simulink model "IEEE9_case"  (R2024b)
settings: Solver=FixedStepAuto  StartTime=0  StopTime=5  FixedStep=1e-7  RelTol=1e-3
values from neighbouring files (symbols this model uses):
  SG_D_1_D = 0.01056    [IEEE9_case_parameters.m]    (also in case1_parameters.m; case2_parameters.m; case3_parameters.m; case4_parameters.m)
  SG_D_1_EnableSaturation = 0    [IEEE9_case_parameters.m]    (also in case1_parameters.m; case2_parameters.m; case3_parameters.m; case4_parameters.m)
  SG_D_1_f0 = 60    [IEEE9_case_parameters.m]    (also in case1_parameters.m; case2_parameters.m; case3_parameters.m; case4_parameters.m)
  SG_D_1_H = 7.5    [IEEE9_case_parameters.m]    (also in case1_parameters.m; case2_parameters.m; case3_parameters.m; case4_parameters.m)
  SG_D_1_K_A = 20    [IEEE9_case_parameters.m]    (also in case1_parameters.m; case2_parameters.m; case3_parameters.m; case4_parameters.m)
  SG_D_1_K_E = 1.000000e+1    (= 10)    [IEEE9_case_parameters.m]    (also in case1_parameters.m; case2_parameters.m; case3_parameters.m; case4_parameters.m)
  SG_D_1_K_F = 2.363    [IEEE9_case_parameters.m]    (also in case1_parameters.m; case2_parameters.m; case3_parameters.m; case4_parameters.m)
  SG_D_1_K_s = 0.5    [IEEE9_case_parameters.m]    (also in case1_parameters.m = 5; case2_parameters.m = 5; case3_parameters.m = 5; case4_parameters.m = 5)
  SG_D_1_R_a = 0.001088    [IEEE9_case_parameters.m]    (also in case1_parameters.m; case2_parameters.m; case3_parameters.m; case4_parameters.m)
  SG_D_1_S_A = 1    [IEEE9_case_parameters.m]    (also in case1_parameters.m; case2_parameters.m; case3_parameters.m; case4_parameters.m)
  SG_D_1_S_B = 0.103    [IEEE9_case_parameters.m]    (also in case1_parameters.m; case2_parameters.m; case3_parameters.m; case4_parameters.m)
  SG_D_1_S_N = 10.659857    [IEEE9_case_parameters.m]    (also in case1_parameters.m; case2_parameters.m; case3_parameters.m; case4_parameters.m)
  SG_D_1_SpeedPara = 200    [IEEE9_case_parameters.m]    (also in case1_parameters.m; case2_parameters.m; case3_parameters.m; case4_parameters.m)
  SG_D_1_T_0 = 0.720173    [IEEE9_case_parameters.m]    (also in case1_parameters.m = 0.755522; case2_parameters.m = 0.808931; case3_parameters.m = 0.869402; case4_parameters.m = 0.729316)
  SG_D_1_T_1 = 0.3    [IEEE9_case_parameters.m]    (also in case1_parameters.m; case2_parameters.m; case3_parameters.m; case4_parameters.m)
  SG_D_1_T_2 = 0.05    [IEEE9_case_parameters.m]    (also in case1_parameters.m; case2_parameters.m; case3_parameters.m; case4_parameters.m)
  SG_D_1_T_3 = 0.02    [IEEE9_case_parameters.m]    (also in case1_parameters.m; case2_parameters.m; case3_parameters.m; case4_parameters.m)
  SG_D_1_T_4 = 0.005    [IEEE9_case_parameters.m]    (also in case1_parameters.m; case2_parameters.m; case3_parameters.m; case4_parameters.m)
  SG_D_1_T_A = 0.02    [IEEE9_case_parameters.m]    (also in case1_parameters.m; case2_parameters.m; case3_parameters.m; case4_parameters.m)
  SG_D_1_T_dd = 8.000000e+0    (= 8)    [IEEE9_case_parameters.m]    (also in case1_parameters.m; case2_parameters.m; case3_parameters.m; case4_parameters.m)
  SG_D_1_T_ddd = 0.04    [IEEE9_case_parameters.m]    (also in case1_parameters.m; case2_parameters.m; case3_parameters.m; case4_parameters.m)
  SG_D_1_T_E = 0.314    [IEEE9_case_parameters.m]    (also in case1_parameters.m; case2_parameters.m; case3_parameters.m; case4_parameters.m)
  SG_D_1_T_F = 0.35    [IEEE9_case_parameters.m]    (also in case1_parameters.m; case2_parameters.m; case3_parameters.m; case4_parameters.m)
  SG_D_1_T_qd = 0.8    [IEEE9_case_parameters.m]    (also in case1_parameters.m; case2_parameters.m; case3_parameters.m; case4_parameters.m)
  SG_D_1_T_qdd = 0.02    [IEEE9_case_parameters.m]    (also in case1_parameters.m; case2_parameters.m; case3_parameters.m; case4_parameters.m)
  SG_D_1_T_speed = 0.1    [IEEE9_case_parameters.m]    (also in case1_parameters.m = 200; case2_parameters.m = 200; case3_parameters.m = 200; case4_parameters.m = 200)
  SG_D_1_T_w = 0.5    [IEEE9_case_parameters.m]    (also in case1_parameters.m; case2_parameters.m; case3_parameters.m; case4_parameters.m)
  SG_D_1_V_ref = 1.990276    [IEEE9_case_parameters.m]    (also in case1_parameters.m = 2.042296; case2_parameters.m = 2.051388; case3_parameters.m = 2.089584; case4_parameters.m = 2.01845)
  SG_D_1_w_ref = 376.991118    [IEEE9_case_parameters.m]    (also in case1_parameters.m; case2_parameters.m; case3_parameters.m; case4_parameters.m)
  SG_D_1_wb = 6.000000e+1    (= 60)    [IEEE9_case_parameters.m]    (also in case1_parameters.m; case2_parameters.m; case3_parameters.m; case4_parameters.m)
  SG_D_1_x_d = 1.9    [IEEE9_case_parameters.m]    (also in case1_parameters.m; case2_parameters.m; case3_parameters.m; case4_parameters.m)
  SG_D_1_x_dd = 0.302    [IEEE9_case_parameters.m]    (also in case1_parameters.m; case2_parameters.m; case3_parameters.m; case4_parameters.m)
  SG_D_1_x_ddd = 0.204    [IEEE9_case_parameters.m]    (also in case1_parameters.m; case2_parameters.m; case3_parameters.m; case4_parameters.m)
  SG_D_1_x_l = 0.05    [IEEE9_case_parameters.m]    (also in case1_parameters.m; case2_parameters.m; case3_parameters.m; case4_parameters.m)
  SG_D_1_x_q = 1.3    [IEEE9_case_parameters.m]    (also in case1_parameters.m; case2_parameters.m; case3_parameters.m; case4_parameters.m)
  SG_D_1_x_qd = 0.5    [IEEE9_case_parameters.m]    (also in case1_parameters.m; case2_parameters.m; case3_parameters.m; case4_parameters.m)
  SG_D_1_x_qdd = 0.3    [IEEE9_case_parameters.m]    (also in case1_parameters.m; case2_parameters.m; case3_parameters.m; case4_parameters.m)
  SG_D_2_D = 0.02    [IEEE9_case_parameters.m]    (also in case1_parameters.m; case2_parameters.m; case3_parameters.m; case4_parameters.m)
  SG_D_2_EnableSaturation = 0    [IEEE9_case_parameters.m]    (also in case1_parameters.m; case2_parameters.m; case3_parameters.m; case4_parameters.m)
  SG_D_2_f0 = 60    [IEEE9_case_parameters.m]    (also in case1_parameters.m; case2_parameters.m; case3_parameters.m; case4_parameters.m)
  SG_D_2_H = 8.000000e+0    (= 8)    [IEEE9_case_parameters.m]    (also in case1_parameters.m; case2_parameters.m; case3_parameters.m; case4_parameters.m)
  SG_D_2_K_A = 20    [IEEE9_case_parameters.m]    (also in case1_parameters.m; case2_parameters.m; case3_parameters.m; case4_parameters.m)
  SG_D_2_K_E = 1.000000e+1    (= 10)    [IEEE9_case_parameters.m]    (also in case1_parameters.m; case2_parameters.m; case3_parameters.m; case4_parameters.m)
  SG_D_2_K_F = 2.363    [IEEE9_case_parameters.m]    (also in case1_parameters.m; case2_parameters.m; case3_parameters.m; case4_parameters.m)
  SG_D_2_K_s = 0.5    [IEEE9_case_parameters.m]    (also in case1_parameters.m = 4; case2_parameters.m = 4; case3_parameters.m = 4; case4_parameters.m = 4)
  SG_D_2_R_a = 0.001088    [IEEE9_case_parameters.m]    (also in case1_parameters.m; case2_parameters.m; case3_parameters.m; case4_parameters.m)
  SG_D_2_S_A = 1    [IEEE9_case_parameters.m]    (also in case1_parameters.m; case2_parameters.m; case3_parameters.m; case4_parameters.m)
  SG_D_2_S_B = 0.103    [IEEE9_case_parameters.m]    (also in case1_parameters.m; case2_parameters.m; case3_parameters.m; case4_parameters.m)
  SG_D_2_S_N = 10.659857    [IEEE9_case_parameters.m]    (also in case1_parameters.m; case2_parameters.m; case3_parameters.m; case4_parameters.m)
  SG_D_2_SpeedPara = 200    [IEEE9_case_parameters.m]    (also in case1_parameters.m; case2_parameters.m; case3_parameters.m; case4_parameters.m)
  SG_D_2_T_0 = 1.632913    [IEEE9_case_parameters.m]    (also in case1_parameters.m = 1.632925; case2_parameters.m = 1.632915; case3_parameters.m = 1.632914; case4_parameters.m = 1.632927)
  SG_D_2_T_1 = 0.2    [IEEE9_case_parameters.m]    (also in case1_parameters.m; case2_parameters.m; case3_parameters.m; case4_parameters.m)
  SG_D_2_T_2 = 0.05    [IEEE9_case_parameters.m]    (also in case1_parameters.m; case2_parameters.m; case3_parameters.m; case4_parameters.m)
  SG_D_2_T_3 = 0.02    [IEEE9_case_parameters.m]    (also in case1_parameters.m; case2_parameters.m; case3_parameters.m; case4_parameters.m)
  SG_D_2_T_4 = 0.005    [IEEE9_case_parameters.m]    (also in case1_parameters.m; case2_parameters.m; case3_parameters.m; case4_parameters.m)
  SG_D_2_T_A = 0.02    [IEEE9_case_parameters.m]    (also in case1_parameters.m; case2_parameters.m; case3_parameters.m; case4_parameters.m)
  SG_D_2_T_dd = 7.9    [IEEE9_case_parameters.m]    (also in case1_parameters.m; case2_parameters.m; case3_parameters.m; case4_parameters.m)
  SG_D_2_T_ddd = 0.04    [IEEE9_case_parameters.m]    (also in case1_parameters.m; case2_parameters.m; case3_parameters.m; case4_parameters.m)
  SG_D_2_T_E = 0.314    [IEEE9_case_parameters.m]    (also in case1_parameters.m; case2_parameters.m; case3_parameters.m; case4_parameters.m)
  SG_D_2_T_F = 0.35    [IEEE9_case_parameters.m]    (also in case1_parameters.m; case2_parameters.m; case3_parameters.m; case4_parameters.m)
  SG_D_2_T_qd = 0.8    [IEEE9_case_parameters.m]    (also in case1_parameters.m; case2_parameters.m; case3_parameters.m; case4_parameters.m)
  SG_D_2_T_qdd = 0.015    [IEEE9_case_parameters.m]    (also in case1_parameters.m; case2_parameters.m; case3_parameters.m; case4_parameters.m)
  SG_D_2_T_speed = 0.1    [IEEE9_case_parameters.m]    (also in case1_parameters.m = 150; case2_parameters.m = 150; case3_parameters.m = 150; case4_parameters.m = 150)
  SG_D_2_T_w = 0.35    [IEEE9_case_parameters.m]    (also in case1_parameters.m; case2_parameters.m; case3_parameters.m; case4_parameters.m)
  SG_D_2_V_ref = 2.58547    [IEEE9_case_parameters.m]    (also in case1_parameters.m = 2.597896; case2_parameters.m = 2.587136; case3_parameters.m = 2.586042; case4_parameters.m = 2.599679)
  SG_D_2_w_ref = 376.991118    [IEEE9_case_parameters.m]    (also in case1_parameters.m; case2_parameters.m; case3_parameters.m; case4_parameters.m)
  SG_D_2_wb = 6.000000e+1    (= 60)    [IEEE9_case_parameters.m]    (also in case1_parameters.m; case2_parameters.m; case3_parameters.m; case4_parameters.m)
  SG_D_2_x_d = 1.8    [IEEE9_case_parameters.m]    (also in case1_parameters.m; case2_parameters.m; case3_parameters.m; case4_parameters.m)
  SG_D_2_x_dd = 0.302    [IEEE9_case_parameters.m]    (also in case1_parameters.m; case2_parameters.m; case3_parameters.m; case4_parameters.m)
  SG_D_2_x_ddd = 0.204    [IEEE9_case_parameters.m]    (also in case1_parameters.m; case2_parameters.m; case3_parameters.m; case4_parameters.m)
  SG_D_2_x_l = 0.05    [IEEE9_case_parameters.m]    (also in case1_parameters.m; case2_parameters.m; case3_parameters.m; case4_parameters.m)
  SG_D_2_x_q = 1.25    [IEEE9_case_parameters.m]    (also in case1_parameters.m; case2_parameters.m; case3_parameters.m; case4_parameters.m)
  SG_D_2_x_qd = 0.5    [IEEE9_case_parameters.m]    (also in case1_parameters.m; case2_parameters.m; case3_parameters.m; case4_parameters.m)
  SG_D_2_x_qdd = 0.3    [IEEE9_case_parameters.m]    (also in case1_parameters.m; case2_parameters.m; case3_parameters.m; case4_parameters.m)
  SG_D_3_D = 0.02    [IEEE9_case_parameters.m]    (also in case1_parameters.m; case2_parameters.m; case3_parameters.m; case4_parameters.m)
  SG_D_3_EnableSaturation = 0    [IEEE9_case_parameters.m]    (also in case1_parameters.m; case2_parameters.m; case3_parameters.m; case4_parameters.m)
  SG_D_3_f0 = 60    [IEEE9_case_parameters.m]    (also in case1_parameters.m; case2_parameters.m; case3_parameters.m; case4_parameters.m)
  SG_D_3_H = 7.7    [IEEE9_case_parameters.m]    (also in case1_parameters.m; case2_parameters.m; case3_parameters.m; case4_parameters.m)
  SG_D_3_K_A = 20    [IEEE9_case_parameters.m]    (also in case1_parameters.m; case2_parameters.m; case3_parameters.m; case4_parameters.m)
  SG_D_3_K_E = 1.000000e+1    (= 10)    [IEEE9_case_parameters.m]    (also in case1_parameters.m; case2_parameters.m; case3_parameters.m; case4_parameters.m)
  SG_D_3_K_F = 2.363    [IEEE9_case_parameters.m]    (also in case1_parameters.m; case2_parameters.m; case3_parameters.m; case4_parameters.m)
  SG_D_3_K_s = 0.2    [IEEE9_case_parameters.m]    (also in case1_parameters.m = 2; case2_parameters.m = 2; case3_parameters.m = 2; case4_parameters.m = 2)
  SG_D_3_R_a = 0.001088    [IEEE9_case_parameters.m]    (also in case1_parameters.m; case2_parameters.m; case3_parameters.m; case4_parameters.m)
  SG_D_3_S_A = 1    [IEEE9_case_parameters.m]    (also in case1_parameters.m; case2_parameters.m; case3_parameters.m; case4_parameters.m)
  SG_D_3_S_B = 0.103    [IEEE9_case_parameters.m]    (also in case1_parameters.m; case2_parameters.m; case3_parameters.m; case4_parameters.m)
  SG_D_3_S_N = 10.659857    [IEEE9_case_parameters.m]    (also in case1_parameters.m; case2_parameters.m; case3_parameters.m; case4_parameters.m)
  SG_D_3_SpeedPara = 200    [IEEE9_case_parameters.m]    (also in case1_parameters.m; case2_parameters.m; case3_parameters.m; case4_parameters.m)
  SG_D_3_T_0 = 0.850788    [IEEE9_case_parameters.m]    (also in case1_parameters.m = 0.850786; case2_parameters.m = 0.850787; case3_parameters.m; case4_parameters.m = 0.850786)
  SG_D_3_T_1 = 0.2    [IEEE9_case_parameters.m]    (also in case1_parameters.m; case2_parameters.m; case3_parameters.m; case4_parameters.m)
  SG_D_3_T_2 = 0.05    [IEEE9_case_parameters.m]    (also in case1_parameters.m; case2_parameters.m; case3_parameters.m; case4_parameters.m)
  SG_D_3_T_3 = 0.02    [IEEE9_case_parameters.m]    (also in case1_parameters.m; case2_parameters.m; case3_parameters.m; case4_parameters.m)
  SG_D_3_T_4 = 0.005    [IEEE9_case_parameters.m]    (also in case1_parameters.m; case2_parameters.m; case3_parameters.m; case4_parameters.m)
  SG_D_3_T_A = 0.02    [IEEE9_case_parameters.m]    (also in case1_parameters.m; case2_parameters.m; case3_parameters.m; case4_parameters.m)
  SG_D_3_T_dd = 8.1    [IEEE9_case_parameters.m]    (also in case1_parameters.m; case2_parameters.m; case3_parameters.m; case4_parameters.m)
  SG_D_3_T_ddd = 0.04    [IEEE9_case_parameters.m]    (also in case1_parameters.m; case2_parameters.m; case3_parameters.m; case4_parameters.m)
  SG_D_3_T_E = 0.314    [IEEE9_case_parameters.m]    (also in case1_parameters.m; case2_parameters.m; case3_parameters.m; case4_parameters.m)
  SG_D_3_T_F = 0.35    [IEEE9_case_parameters.m]    (also in case1_parameters.m; case2_parameters.m; case3_parameters.m; case4_parameters.m)
  SG_D_3_T_qd = 0.8    [IEEE9_case_parameters.m]    (also in case1_parameters.m; case2_parameters.m; case3_parameters.m; case4_parameters.m)
  SG_D_3_T_qdd = 0.015    [IEEE9_case_parameters.m]    (also in case1_parameters.m; case2_parameters.m; case3_parameters.m; case4_parameters.m)
  SG_D_3_T_speed = 0.1    [IEEE9_case_parameters.m]    (also in case1_parameters.m = 180; case2_parameters.m = 180; case3_parameters.m = 180; case4_parameters.m = 180)
  SG_D_3_T_w = 0.4    [IEEE9_case_parameters.m]    (also in case1_parameters.m; case2_parameters.m; case3_parameters.m; case4_parameters.m)
  SG_D_3_V_ref = 1.892727    [IEEE9_case_parameters.m]    (also in case1_parameters.m = 1.906439; case2_parameters.m = 1.895535; case3_parameters.m = 1.892105; case4_parameters.m = 1.906598)
  SG_D_3_w_ref = 376.991118    [IEEE9_case_parameters.m]    (also in case1_parameters.m; case2_parameters.m; case3_parameters.m; case4_parameters.m)
  SG_D_3_wb = 6.000000e+1    (= 60)    [IEEE9_case_parameters.m]    (also in case1_parameters.m; case2_parameters.m; case3_parameters.m; case4_parameters.m)
  SG_D_3_x_d = 1.85    [IEEE9_case_parameters.m]    (also in case1_parameters.m; case2_parameters.m; case3_parameters.m; case4_parameters.m)
  SG_D_3_x_dd = 0.302    [IEEE9_case_parameters.m]    (also in case1_parameters.m; case2_parameters.m; case3_parameters.m; case4_parameters.m)
  SG_D_3_x_ddd = 0.204    [IEEE9_case_parameters.m]    (also in case1_parameters.m; case2_parameters.m; case3_parameters.m; case4_parameters.m)
  SG_D_3_x_l = 0.05    [IEEE9_case_parameters.m]    (also in case1_parameters.m; case2_parameters.m; case3_parameters.m; case4_parameters.m)
  SG_D_3_x_q = 1.2    [IEEE9_case_parameters.m]    (also in case1_parameters.m; case2_parameters.m; case3_parameters.m; case4_parameters.m)
  SG_D_3_x_qd = 0.5    [IEEE9_case_parameters.m]    (also in case1_parameters.m; case2_parameters.m; case3_parameters.m; case4_parameters.m)
  SG_D_3_x_qdd = 0.3    [IEEE9_case_parameters.m]    (also in case1_parameters.m; case2_parameters.m; case3_parameters.m; case4_parameters.m)
(part 6 of 12)

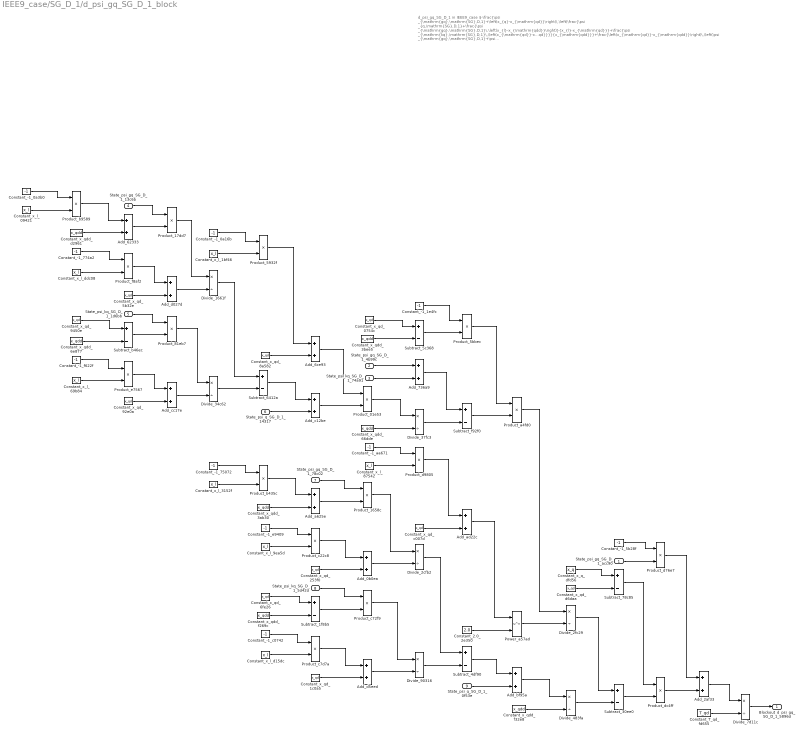
== system IEEE9_case/SG_D_1/d_psi_gq_SG_D_1_block ==
  note: d_psi_gq_SG_D_1 in IEEE9_case
      | $-\frac{\psi _{\mathrm{gq},\mathrm{SG},D,1}+\left(x_{q}-x_{\mathrm{qd}}\right)\,\left(\frac{\psi _{q,\mathrm{SG},D,1}+\frac{\psi _{\mathrm{gq},\mathrm{SG},D,1}\,\left(x_{l}-x_{\mathrm{qdd}}\right)}{x_{l}-x_{\mathrm{qd}}}+\frac{\psi _{\mathrm{kq},\mathrm{SG},D,1}\,\left(x_{\mathrm{qd}}-x_{\mathrm{qdd}}\right)}{x_{l}-x_{\mathrm{qd}}}}{x_{\mathrm{qdd}}}+\frac{\left(x_{\mathrm{qd}}-x_{\mathrm{qdd}}\right)\,\left(\psi _{\mathrm{gq},\mathrm{SG},D,1}+\psi _{\mathrm{kq},\mathrm{SG},D,1}+\frac{\left(x_{l}-x_{\mathrm{qd}}\right)\,\left(\psi _{q,\mathrm{SG},D,1}+\frac{\psi _{\mathrm{gq},\mathrm{SG},D,1}\,\left(x_{l}-x_{\mathrm{qdd}}\right)}{x_{l}-x_{\mathrm{qd}}}+\frac{\psi _{\mathrm{kq},\mathrm{SG},D,1}\,\left(x_{\mathrm{qd}}-x_{\mathrm{qdd}}\right)}{x_{l}-x_{\mathrm{qd}}}\right)}{x_{\mathrm{qdd}}}\right)}{{\left(x_{l}-x_{\mathrm{qd}}\right)}^2}\right)}{T_{\mathrm{qd}}}$
      | Automatically generated on 2025-11-01 08:47:44 .
  State_psi_gq_SG_D_1_acc90 : Inport
  State_psi_gq_SG_D_1_4b99c : Inport  Port=2
  State_psi_kq_SG_D_1_74a91 : Inport  Port=3
  State_psi_gq_SG_D_1_13c6b : Inport  Port=4
  State_psi_kq_SG_D_1_1d6bb : Inport  Port=5
  State_psi_q_SG_D_1_14317 : Inport  Port=6
  State_psi_gq_SG_D_1_78c02 : Inport  Port=7
  State_psi_kq_SG_D_1_5d42d : Inport  Port=8
  State_psi_q_SG_D_1_0f53e : Inport  Port=9
  Add_0b0ea : Sum
  Add_2af33 : Sum
  Add_62333 : Sum
  Add_6ce93 : Sum
  Add_736a9 : Sum
  Add_a625e : Sum
  Add_ad22c : Sum
  Add_bf95a : Sum
  Add_c12be : Sum
  Add_cc17e : Sum
  Add_d027d : Sum
  Add_d5eed : Sum
  Constant_-1_0a16b : Constant  Value=-1
  Constant_-1_0a3b0 : Constant  Value=-1
  Constant_-1_1e4fc : Constant  Value=-1
  Constant_-1_5b28f : Constant  Value=-1
  Constant_-1_75072 : Constant  Value=-1
  Constant_-1_774a2 : Constant  Value=-1
  Constant_-1_aa671 : Constant  Value=-1
  Constant_-1_c0742 : Constant  Value=-1
  Constant_-1_e9409 : Constant  Value=-1
  Constant_-1_f622f : Constant  Value=-1
  Constant_2.0_2e350 : Constant  Value=2.0
  Constant_T_qd_fd655 : Constant  Value=T_qd
  Constant_x_l_09421 : Constant  Value=x_l
  Constant_x_l_1bf46 : Constant  Value=x_l
  Constant_x_l_3152f : Constant  Value=x_l
  Constant_x_l_69b84 : Constant  Value=x_l
  Constant_x_l_87542 : Constant  Value=x_l
  Constant_x_l_9ea5d : Constant  Value=x_l
  Constant_x_l_d15dc : Constant  Value=x_l
  Constant_x_l_ddc08 : Constant  Value=x_l
  Constant_x_q_dfd56 : Constant  Value=x_q
  Constant_x_qd_0754c : Constant  Value=x_qd
  Constant_x_qd_1c0a5 : Constant  Value=x_qd
  Constant_x_qd_253f0 : Constant  Value=x_qd
  Constant_x_qd_5b32e : Constant  Value=x_qd
  Constant_x_qd_6fe26 : Constant  Value=x_qd
  Constant_x_qd_8a582 : Constant  Value=x_qd
  Constant_x_qd_92e0a : Constant  Value=x_qd
  Constant_x_qd_9450e : Constant  Value=x_qd
  Constant_x_qd_c007d : Constant  Value=x_qd
  Constant_x_qd_d6daa : Constant  Value=x_qd
  Constant_x_qdd_3ab30 : Constant  Value=x_qdd
  Constant_x_qdd_3bee5 : Constant  Value=x_qdd
  Constant_x_qdd_66dde : Constant  Value=x_qdd
  Constant_x_qdd_6e877 : Constant  Value=x_qdd
  Constant_x_qdd_d2961 : Constant  Value=x_qdd
  Constant_x_qdd_f269c : Constant  Value=x_qdd
  Constant_x_qdd_f32e8 : Constant  Value=x_qdd
  Divide_1661f : Product  Inputs=*/
  Divide_2cfb2 : Product  Inputs=*/
  Divide_2fc29 : Product  Inputs=*/
  Divide_34c62 : Product  Inputs=*/
  Divide_37fc3 : Product  Inputs=*/
  Divide_483fa : Product  Inputs=*/
  Divide_7d11c : Product  Inputs=*/
  Divide_90316 : Product  Inputs=*/
  Power_a57ad : Math  Operator=pow
  Product_01e53 : Product
  Product_1658c : Product
  Product_17dd7 : Product
  Product_5932f : Product
  Product_5bbec : Product
  Product_81eb7 : Product
  Product_a4fd0 : Product
  Product_b435c : Product
  Product_b9589 : Product
  Product_c22c8 : Product
  Product_c72f9 : Product
  Product_c7d7a : Product
  Product_d76e7 : Product
  Product_d9805 : Product
  Product_dc4ff : Product
  Product_e7567 : Product
  Product_f8af2 : Product
  Subtract_1f8b5 : Sum  Inputs=+-
  Subtract_30ee0 : Sum  Inputs=+-
  Subtract_4df90 : Sum  Inputs=+-
  Subtract_5c368 : Sum  Inputs=+-
  Subtract_6412a : Sum  Inputs=+-
  Subtract_78c85 : Sum  Inputs=+-
  Subtract_b46ec : Sum  Inputs=+-
  Subtract_f92f0 : Sum  Inputs=+-
  Blockout_d_psi_gq_SG_D_1_5896d : Outport
  wires:
  State_psi_gq_SG_D_1_13c6b/1 -> Product_17dd7/1
  Constant_-1_774a2/1 -> Product_f8af2/1
  Divide_1661f/1 -> Subtract_6412a/1
  Add_d027d/1 -> Divide_1661f/2
  Product_b9589/1 -> Add_62333/1
  Constant_x_qd_8a582/1 -> Add_6ce93/2
  Constant_-1_0a3b0/1 -> Product_b9589/1
  Constant_x_qdd_d2961/1 -> Add_62333/2
  Constant_x_l_ddc08/1 -> Product_f8af2/2
  Constant_x_l_09421/1 -> Product_b9589/2
  Constant_-1_f622f/1 -> Product_e7567/1
  Constant_x_qd_9450e/1 -> Subtract_b46ec/1
  Constant_x_qdd_66dde/1 -> Divide_37fc3/2
  Constant_x_l_69b84/1 -> Product_e7567/2
  Constant_x_qdd_6e877/1 -> Subtract_b46ec/2
  Subtract_6412a/1 -> Add_c12be/1
  Add_62333/1 -> Product_17dd7/2
  Product_17dd7/1 -> Divide_1661f/1
  Product_f8af2/1 -> Add_d027d/1
  Constant_x_qd_5b32e/1 -> Add_d027d/2
  State_psi_kq_SG_D_1_1d6bb/1 -> Product_81eb7/1
  Product_e7567/1 -> Add_cc17e/1
  Subtract_b46ec/1 -> Product_81eb7/2
  Constant_x_qd_92e0a/1 -> Add_cc17e/2
  Product_81eb7/1 -> Divide_34c62/1
  Add_cc17e/1 -> Divide_34c62/2
  Constant_-1_1e4fc/1 -> Product_5bbec/1
  Constant_-1_0a16b/1 -> Product_5932f/1
  Add_0b0ea/1 -> Divide_2cfb2/2
  Product_c7d7a/1 -> Add_d5eed/1
  Subtract_1f8b5/1 -> Product_c72f9/2
  Constant_x_l_1bf46/1 -> Product_5932f/2
  Divide_34c62/1 -> Subtract_6412a/2
  Subtract_78c85/1 -> Product_dc4ff/1
  Constant_-1_aa671/1 -> Product_d9805/1
  Constant_-1_75072/1 -> Product_b435c/1
  Constant_x_l_87542/1 -> Product_d9805/2
  Constant_x_l_3152f/1 -> Product_b435c/2
  Constant_x_qd_253f0/1 -> Add_0b0ea/2
  Product_5932f/1 -> Add_6ce93/1
  State_psi_q_SG_D_1_14317/1 -> Add_c12be/2
  Product_b435c/1 -> Add_a625e/1
  Constant_x_qdd_3ab30/1 -> Add_a625e/2
  Constant_-1_e9409/1 -> Product_c22c8/1
  Constant_x_qd_1c0a5/1 -> Add_d5eed/2
  Add_6ce93/1 -> Product_01e53/1
  Constant_x_l_9ea5d/1 -> Product_c22c8/2
  Constant_-1_c0742/1 -> Product_c7d7a/1
  Constant_x_qd_6fe26/1 -> Subtract_1f8b5/1
  Product_01e53/1 -> Divide_37fc3/1
  Constant_x_l_d15dc/1 -> Product_c7d7a/2
  Divide_2fc29/1 -> Subtract_30ee0/1
  Constant_x_qdd_f269c/1 -> Subtract_1f8b5/2
  Add_c12be/1 -> Product_01e53/2
  State_psi_gq_SG_D_1_78c02/1 -> Product_1658c/1
  Add_a625e/1 -> Product_1658c/2
  Product_c22c8/1 -> Add_0b0ea/1
  State_psi_kq_SG_D_1_5d42d/1 -> Product_c72f9/1
  Add_d5eed/1 -> Divide_90316/2
  State_psi_gq_SG_D_1_4b99c/1 -> Add_736a9/1
  Constant_x_qd_0754c/1 -> Subtract_5c368/1
  Constant_x_qdd_3bee5/1 -> Subtract_5c368/2
  Product_c72f9/1 -> Divide_90316/1
  State_psi_kq_SG_D_1_74a91/1 -> Add_736a9/2
  Product_1658c/1 -> Divide_2cfb2/1
  Subtract_5c368/1 -> Product_5bbec/2
  Add_736a9/1 -> Subtract_f92f0/1
  Divide_37fc3/1 -> Subtract_f92f0/2
  Product_d9805/1 -> Add_ad22c/1
  Constant_x_qd_c007d/1 -> Add_ad22c/2
  Divide_2cfb2/1 -> Subtract_4df90/1
  Divide_90316/1 -> Subtract_4df90/2
  Product_5bbec/1 -> Product_a4fd0/1
  Subtract_f92f0/1 -> Product_a4fd0/2
  Add_ad22c/1 -> Power_a57ad/1
  Constant_2.0_2e350/1 -> Power_a57ad/2
  Subtract_4df90/1 -> Add_bf95a/1
  State_psi_q_SG_D_1_0f53e/1 -> Add_bf95a/2
  Product_a4fd0/1 -> Divide_2fc29/1
  Power_a57ad/1 -> Divide_2fc29/2
  Add_bf95a/1 -> Divide_483fa/1
  Constant_x_qdd_f32e8/1 -> Divide_483fa/2
  Constant_x_q_dfd56/1 -> Subtract_78c85/1
  Constant_x_qd_d6daa/1 -> Subtract_78c85/2
  Divide_483fa/1 -> Subtract_30ee0/2
  Constant_-1_5b28f/1 -> Product_d76e7/1
  State_psi_gq_SG_D_1_acc90/1 -> Product_d76e7/2
  Subtract_30ee0/1 -> Product_dc4ff/2
  Product_d76e7/1 -> Add_2af33/1
  Product_dc4ff/1 -> Add_2af33/2
  Add_2af33/1 -> Divide_7d11c/1
  Constant_T_qd_fd655/1 -> Divide_7d11c/2
  Divide_7d11c/1 -> Blockout_d_psi_gq_SG_D_1_5896d/1

== system IEEE9_case/SG_D_1/d_psi_kq_SG_D_1_block ==
  note: d_psi_kq_SG_D_1 in IEEE9_case
      | $-\frac{\psi _{\mathrm{gq},\mathrm{SG},D,1}+\psi _{\mathrm{kq},\mathrm{SG},D,1}+\frac{\left(x_{l}-x_{\mathrm{qd}}\right)\,\left(\psi _{q,\mathrm{SG},D,1}+\frac{\psi _{\mathrm{gq},\mathrm{SG},D,1}\,\left(x_{l}-x_{\mathrm{qdd}}\right)}{x_{l}-x_{\mathrm{qd}}}+\frac{\psi _{\mathrm{kq},\mathrm{SG},D,1}\,\left(x_{\mathrm{qd}}-x_{\mathrm{qdd}}\right)}{x_{l}-x_{\mathrm{qd}}}\right)}{x_{\mathrm{qdd}}}}{T_{\mathrm{qdd}}}$
      | Automatically generated on 2025-11-01 08:47:48 .
  State_psi_gq_SG_D_1_49d8b : Inport
  State_psi_kq_SG_D_1_01b22 : Inport  Port=2
  State_psi_gq_SG_D_1_47bd3 : Inport  Port=3
  State_psi_kq_SG_D_1_dfcd5 : Inport  Port=4
  State_psi_q_SG_D_1_68fd5 : Inport  Port=5
  Add_084c3 : Sum
  Add_2c012 : Sum
  Add_2f0c8 : Sum
  Add_49d96 : Sum
  Add_85ea5 : Sum
  Add_fad76 : Sum
  Constant_-1_72ab9 : Constant  Value=-1
  Constant_-1_92c62 : Constant  Value=-1
  Constant_-1_ac321 : Constant  Value=-1
  Constant_-1_b5108 : Constant  Value=-1
  Constant_-1_c3780 : Constant  Value=-1
  Constant_T_qdd_57beb : Constant  Value=T_qdd
  Constant_x_l_311b0 : Constant  Value=x_l
  Constant_x_l_3981a : Constant  Value=x_l
  Constant_x_l_62966 : Constant  Value=x_l
  Constant_x_l_98c38 : Constant  Value=x_l
  Constant_x_qd_3af05 : Constant  Value=x_qd
  Constant_x_qd_6fbee : Constant  Value=x_qd
  Constant_x_qd_a7fbb : Constant  Value=x_qd
  Constant_x_qd_cbc91 : Constant  Value=x_qd
  Constant_x_qdd_0a2c9 : Constant  Value=x_qdd
  Constant_x_qdd_25906 : Constant  Value=x_qdd
  Constant_x_qdd_e3520 : Constant  Value=x_qdd
  Divide_1a1ce : Product  Inputs=*/
  Divide_5f60d : Product  Inputs=*/
  Divide_7895a : Product  Inputs=*/
  Divide_f11d6 : Product  Inputs=*/
  Product_0ea38 : Product
  Product_3e32f : Product
  Product_40f55 : Product
  Product_67d0d : Product
  Product_b6550 : Product
  Product_c92d2 : Product
  Product_cd562 : Product
  Product_d66a1 : Product
  Subtract_0bd57 : Sum  Inputs=+-
  Subtract_bee95 : Sum  Inputs=+-
  Subtract_e02f6 : Sum  Inputs=+-
  Blockout_d_psi_kq_SG_D_1_c4f81 : Outport
  wires:
  Product_d66a1/1 -> Add_084c3/1
  Constant_-1_72ab9/1 -> Product_d66a1/1
  Constant_x_l_62966/1 -> Product_d66a1/2
  Constant_x_qdd_0a2c9/1 -> Add_084c3/2
  Constant_-1_92c62/1 -> Product_c92d2/1
  Constant_x_qd_6fbee/1 -> Subtract_e02f6/1
  Constant_x_qd_cbc91/1 -> Add_49d96/2
  Constant_-1_ac321/1 -> Product_40f55/1
  Constant_x_l_98c38/1 -> Product_c92d2/2
  Constant_x_qdd_25906/1 -> Subtract_e02f6/2
  Constant_x_qd_a7fbb/1 -> Add_2f0c8/2
  Constant_x_l_3981a/1 -> Product_40f55/2
  Subtract_bee95/1 -> Add_fad76/1
  Product_67d0d/1 -> Subtract_bee95/1
  State_psi_gq_SG_D_1_47bd3/1 -> Product_cd562/1
  Add_084c3/1 -> Product_cd562/2
  Product_40f55/1 -> Add_85ea5/1
  Constant_x_qd_3af05/1 -> Add_85ea5/2
  State_psi_kq_SG_D_1_dfcd5/1 -> Product_0ea38/1
  Product_c92d2/1 -> Add_2f0c8/1
  Subtract_e02f6/1 -> Product_0ea38/2
  Product_cd562/1 -> Divide_7895a/1
  Add_85ea5/1 -> Divide_7895a/2
  Product_0ea38/1 -> Divide_f11d6/1
  Add_2f0c8/1 -> Divide_f11d6/2
  Constant_-1_c3780/1 -> Product_3e32f/1
  Constant_x_l_311b0/1 -> Product_3e32f/2
  Divide_7895a/1 -> Subtract_0bd57/1
  Divide_f11d6/1 -> Subtract_0bd57/2
  Product_3e32f/1 -> Add_49d96/1
  Add_2c012/1 -> Product_b6550/2
  Subtract_0bd57/1 -> Add_2c012/1
  State_psi_q_SG_D_1_68fd5/1 -> Add_2c012/2
  Constant_-1_b5108/1 -> Product_67d0d/1
  State_psi_gq_SG_D_1_49d8b/1 -> Product_67d0d/2
  Divide_5f60d/1 -> Add_fad76/2
  Product_b6550/1 -> Divide_5f60d/1
  Add_49d96/1 -> Product_b6550/1
  State_psi_kq_SG_D_1_01b22/1 -> Subtract_bee95/2
  Constant_x_qdd_e3520/1 -> Divide_5f60d/2
  Add_fad76/1 -> Divide_1a1ce/1
  Constant_T_qdd_57beb/1 -> Divide_1a1ce/2
  Divide_1a1ce/1 -> Blockout_d_psi_kq_SG_D_1_c4f81/1

== system IEEE9_case/SG_D_1/d_psi_q_SG_D_1_block ==
  note: d_psi_q_SG_D_1 in IEEE9_case
      | $2\,\pi \,f_{0}\,\left(v_{d,\mathrm{SG},D,1}\,\cos\left(\theta _{\mathrm{SG},D,1}\right)+v_{q,\mathrm{SG},D,1}\,\sin\left(\theta _{\mathrm{SG},D,1}\right)-\frac{R_{a}\,\left(\psi _{q,\mathrm{SG},D,1}+\frac{\psi _{\mathrm{gq},\mathrm{SG},D,1}\,\left(x_{l}-x_{\mathrm{qdd}}\right)}{x_{l}-x_{\mathrm{qd}}}+\frac{\psi _{\mathrm{kq},\mathrm{SG},D,1}\,\left(x_{\mathrm{qd}}-x_{\mathrm{qdd}}\right)}{x_{l}-x_{\mathrm{qd}}}\right)}{x_{\mathrm{qdd}}}-\frac{\psi _{d,\mathrm{SG},D,1}\,w_{\mathrm{SG},D,1}}{2\,f_{0}\,\pi }\right)$
      | Automatically generated on 2025-11-01 08:47:30 .
  State_psi_gq_SG_D_1_fe9b5 : Inport
  State_psi_kq_SG_D_1_3d651 : Inport  Port=2
  State_psi_q_SG_D_1_a2647 : Inport  Port=3
  Input_v_d_SG_D_1_aa1d3 : Inport  Port=4
  State_theta_SG_D_1_e1395 : Inport  Port=5
  Input_v_q_SG_D_1_6253c : Inport  Port=6
  State_theta_SG_D_1_1d708 : Inport  Port=7
  State_psi_d_SG_D_1_0e471 : Inport  Port=8
  State_w_SG_D_1_e9f82 : Inport  Port=9
  Add_64164 : Sum
  Add_8537b : Sum
  Add_a3bc7 : Sum
  Add_e4100 : Sum
  Add_f3d78 : Sum
  Constant_-1_378a8 : Constant  Value=-1
  Constant_-1_8133f : Constant  Value=-1
  Constant_-1_824a9 : Constant  Value=-1
  Constant_-2.0_f55fb : Constant  Value=-2.0
  Constant_2.0_8d344 : Constant  Value=2.0
  Constant_R_a_47c19 : Constant  Value=R_a
  Constant_f0_008b0 : Constant  Value=f0
  Constant_f0_d762c : Constant  Value=f0
  Constant_pi_88ed3 : Constant  Value=pi
  Constant_pi_b8582 : Constant  Value=pi
  Constant_x_l_75fd0 : Constant  Value=x_l
  Constant_x_l_9272e : Constant  Value=x_l
  Constant_x_l_d1231 : Constant  Value=x_l
  Constant_x_qd_31a16 : Constant  Value=x_qd
  Constant_x_qd_99915 : Constant  Value=x_qd
  Constant_x_qd_ddfde : Constant  Value=x_qd
  Constant_x_qdd_79635 : Constant  Value=x_qdd
  Constant_x_qdd_9692b : Constant  Value=x_qdd
  Constant_x_qdd_e0a52 : Constant  Value=x_qdd
  Divide_26b18 : Product  Inputs=*/
  Divide_58e0c : Product  Inputs=*/
  Divide_db486 : Product  Inputs=*/
  Divide_f4fda : Product  Inputs=*/
  MathFunc_cos_7413d : Trigonometry  Operator=cos
  MathFunc_sin_d5432 : Trigonometry
  Product_1b898 : Product
  Product_222a6 : Product
  Product_23150 : Product
  Product_38373 : Product
  Product_4e977 : Product
  Product_5d213 : Product
  Product_85cbe : Product
  Product_9491a : Product
  Product_ac05d : Product
  Product_ac7c1 : Product
  Product_c7f19 : Product
  Product_e3c16 : Product
  Product_e50f5 : Product
  Product_f3949 : Product
  Subtract_0b327 : Sum  Inputs=+-
  Subtract_2a20b : Sum  Inputs=+-
  Subtract_33392 : Sum  Inputs=+-
  Subtract_d7ddd : Sum  Inputs=+-
  Blockout_d_psi_q_SG_D_1_5ed42 : Outport
  wires:
  Divide_26b18/1 -> Subtract_2a20b/1
  Product_e50f5/1 -> Add_64164/1
  Constant_x_l_75fd0/1 -> Product_e50f5/2
  Constant_-1_378a8/1 -> Product_e50f5/1
  Constant_x_qdd_e0a52/1 -> Add_64164/2
  Constant_x_l_d1231/1 -> Product_5d213/2
  Constant_-1_824a9/1 -> Product_5d213/1
  Constant_x_l_9272e/1 -> Product_c7f19/2
  Constant_x_qdd_9692b/1 -> Subtract_0b327/2
  State_psi_kq_SG_D_1_3d651/1 -> Product_ac7c1/1
  Constant_-1_8133f/1 -> Product_c7f19/1
  Constant_x_qd_31a16/1 -> Subtract_0b327/1
  State_psi_gq_SG_D_1_fe9b5/1 -> Product_f3949/1
  Product_1b898/1 -> Blockout_d_psi_q_SG_D_1_5ed42/1
  Subtract_2a20b/1 -> Add_8537b/1
  Product_f3949/1 -> Divide_26b18/1
  Add_64164/1 -> Product_f3949/2
  Divide_f4fda/1 -> Subtract_2a20b/2
  Product_5d213/1 -> Add_f3d78/1
  Constant_x_qd_ddfde/1 -> Add_f3d78/2
  Constant_-2.0_f55fb/1 -> Product_ac05d/1
  Product_ac7c1/1 -> Divide_f4fda/1
  Product_c7f19/1 -> Add_e4100/1
  Subtract_0b327/1 -> Product_ac7c1/2
  Constant_x_qd_99915/1 -> Add_e4100/2
  Add_f3d78/1 -> Divide_26b18/2
  Add_e4100/1 -> Divide_f4fda/2
  Constant_f0_008b0/1 -> Product_38373/2
  State_psi_q_SG_D_1_a2647/1 -> Add_8537b/2
  Product_9491a/1 -> Product_85cbe/1
  Constant_R_a_47c19/1 -> Product_23150/1
  Product_85cbe/1 -> Divide_db486/2
  Product_23150/1 -> Divide_58e0c/1
  Add_8537b/1 -> Product_23150/2
  State_theta_SG_D_1_e1395/1 -> MathFunc_cos_7413d/1
  Input_v_d_SG_D_1_aa1d3/1 -> Product_222a6/1
  Constant_x_qdd_79635/1 -> Divide_58e0c/2
  MathFunc_cos_7413d/1 -> Product_222a6/2
  State_theta_SG_D_1_1d708/1 -> MathFunc_sin_d5432/1
  Divide_58e0c/1 -> Subtract_d7ddd/1
  Constant_2.0_8d344/1 -> Product_9491a/1
  State_w_SG_D_1_e9f82/1 -> Product_4e977/2
  Constant_pi_88ed3/1 -> Product_9491a/2
  Subtract_33392/1 -> Add_a3bc7/1
  Product_222a6/1 -> Subtract_d7ddd/2
  Divide_db486/1 -> Add_a3bc7/2
  Input_v_q_SG_D_1_6253c/1 -> Product_e3c16/1
  MathFunc_sin_d5432/1 -> Product_e3c16/2
  Product_e3c16/1 -> Subtract_33392/2
  State_psi_d_SG_D_1_0e471/1 -> Product_4e977/1
  Constant_f0_d762c/1 -> Product_85cbe/2
  Constant_pi_b8582/1 -> Product_ac05d/2
  Subtract_d7ddd/1 -> Subtract_33392/1
  Product_4e977/1 -> Divide_db486/1
  Product_ac05d/1 -> Product_38373/1
  Product_38373/1 -> Product_1b898/1
  Add_a3bc7/1 -> Product_1b898/2

== system IEEE9_case/SG_D_1/d_theta_SG_D_1_block ==
  note: d_theta_SG_D_1 in IEEE9_case
      | $w_{\mathrm{SG},D,1}-2\,\pi \,f_{0}$
      | Automatically generated on 2025-11-01 08:47:54 .
  State_w_SG_D_1_6c997 : Inport
  Add_edccc : Sum
  Constant_-2.0_cad52 : Constant  Value=-2.0
  Constant_f0_90647 : Constant  Value=f0
  Constant_pi_08232 : Constant  Value=pi
  Product_12d3a : Product
  Product_b4595 : Product
  Blockout_d_theta_SG_D_1_678a9 : Outport
  wires:
  State_w_SG_D_1_6c997/1 -> Add_edccc/2
  Constant_-2.0_cad52/1 -> Product_b4595/1
  Constant_f0_90647/1 -> Product_12d3a/2
  Constant_pi_08232/1 -> Product_b4595/2
  Product_12d3a/1 -> Add_edccc/1
  Product_b4595/1 -> Product_12d3a/1
  Add_edccc/1 -> Blockout_d_theta_SG_D_1_678a9/1

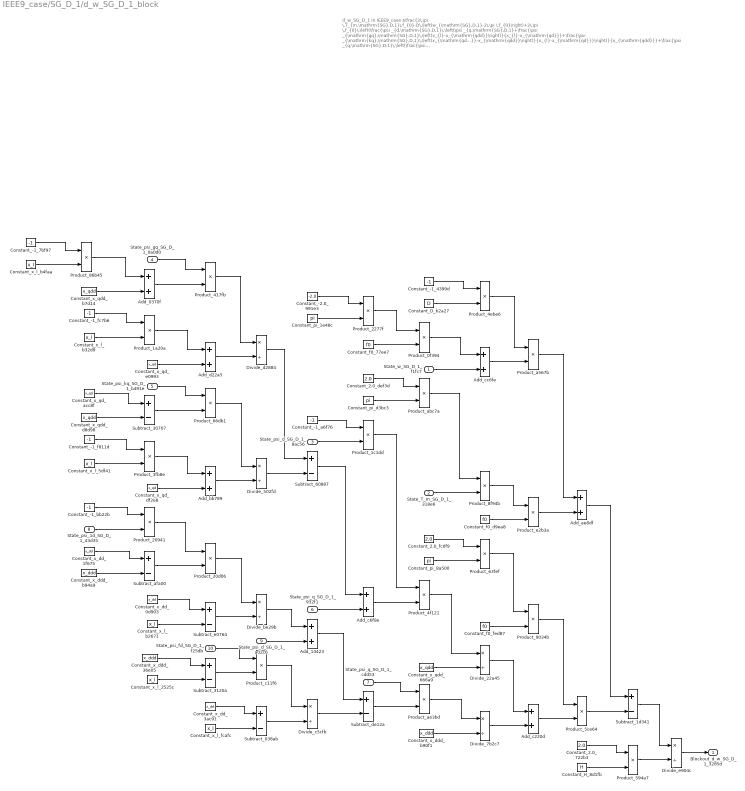
== system IEEE9_case/SG_D_1/d_w_SG_D_1_block ==
  note: d_w_SG_D_1 in IEEE9_case
      | $\frac{2\,\pi \,T_{m,\mathrm{SG},D,1}\,f_{0}-D\,\left(w_{\mathrm{SG},D,1}-2\,\pi \,f_{0}\right)+2\,\pi \,f_{0}\,\left(\frac{\psi _{d,\mathrm{SG},D,1}\,\left(\psi _{q,\mathrm{SG},D,1}+\frac{\psi _{\mathrm{gq},\mathrm{SG},D,1}\,\left(x_{l}-x_{\mathrm{qdd}}\right)}{x_{l}-x_{\mathrm{qd}}}+\frac{\psi _{\mathrm{kq},\mathrm{SG},D,1}\,\left(x_{\mathrm{qd}}-x_{\mathrm{qdd}}\right)}{x_{l}-x_{\mathrm{qd}}}\right)}{x_{\mathrm{qdd}}}+\frac{\psi _{q,\mathrm{SG},D,1}\,\left(\frac{\psi _{\mathrm{1d},\mathrm{SG},D,1}\,\left(x_{\mathrm{dd}}-x_{\mathrm{ddd}}\right)}{x_{\mathrm{dd}}-x_{l}}-\psi _{d,\mathrm{SG},D,1}+\frac{\psi _{\mathrm{fd},\mathrm{SG},D,1}\,\left(x_{\mathrm{ddd}}-x_{l}\right)}{x_{\mathrm{dd}}-x_{l}}\right)}{x_{\mathrm{ddd}}}\right)}{2\,H}$
      | Automatically generated on 2025-11-01 08:47:53 .
  State_w_SG_D_1_f1fc7 : Inport
  State_T_m_SG_D_1_318e6 : Inport  Port=2
  State_psi_d_SG_D_1_8ac56 : Inport  Port=3
  State_psi_gq_SG_D_1_0a0d0 : Inport  Port=4
  State_psi_kq_SG_D_1_b491e : Inport  Port=5
  State_psi_q_SG_D_1_932f1 : Inport  Port=6
  State_psi_q_SG_D_1_cdd53 : Inport  Port=7
  State_psi_1d_SG_D_1_43d35 : Inport  Port=8
  State_psi_d_SG_D_1_a02c6 : Inport  Port=9
  State_psi_fd_SG_D_1_f25db : Inport  Port=10
  Add_0370f : Sum
  Add_14423 : Sum
  Add_ae8df : Sum
  Add_bb789 : Sum
  Add_c220d : Sum
  Add_c6f8e : Sum
  Add_cc6fe : Sum
  Add_d22a5 : Sum
  Constant_-1_4399d : Constant  Value=-1
  Constant_-1_7bf97 : Constant  Value=-1
  Constant_-1_a6f76 : Constant  Value=-1
  Constant_-1_bb22b : Constant  Value=-1
  Constant_-1_f811d : Constant  Value=-1
  Constant_-1_fc7b6 : Constant  Value=-1
  Constant_-2.0_991e3 : Constant  Value=-2.0
  Constant_2.0_722b3 : Constant  Value=2.0
  Constant_2.0_def3d : Constant  Value=2.0
  Constant_2.0_fc0f9 : Constant  Value=2.0
  Constant_D_b2a27 : Constant  Value=D
  Constant_H_8d1fb : Constant  Value=H
  Constant_f0_77ee7 : Constant  Value=f0
  Constant_f0_d9ea8 : Constant  Value=f0
  Constant_f0_fed87 : Constant  Value=f0
  Constant_pi_1e48c : Constant  Value=pi
  Constant_pi_8a500 : Constant  Value=pi
  Constant_pi_d3bc3 : Constant  Value=pi
  Constant_x_dd_0d903 : Constant  Value=x_dd
  Constant_x_dd_1f675 : Constant  Value=x_dd
  Constant_x_dd_3ac91 : Constant  Value=x_dd
  Constant_x_ddd_36e05 : Constant  Value=x_ddd
  Constant_x_ddd_b90f1 : Constant  Value=x_ddd
  Constant_x_ddd_b94a9 : Constant  Value=x_ddd
  Constant_x_l_2525c : Constant  Value=x_l
  Constant_x_l_5df41 : Constant  Value=x_l
  Constant_x_l_b2671 : Constant  Value=x_l
  Constant_x_l_b32d9 : Constant  Value=x_l
  Constant_x_l_b4faa : Constant  Value=x_l
  Constant_x_l_fcafc : Constant  Value=x_l
  Constant_x_qd_acc8f : Constant  Value=x_qd
  Constant_x_qd_df2e8 : Constant  Value=x_qd
  Constant_x_qd_e0993 : Constant  Value=x_qd
  Constant_x_qdd_666a9 : Constant  Value=x_qdd
  Constant_x_qdd_b7d14 : Constant  Value=x_qdd
  Constant_x_qdd_d8d98 : Constant  Value=x_qdd
  Divide_22a45 : Product  Inputs=*/
  Divide_502fd : Product  Inputs=*/
  Divide_7b2c7 : Product  Inputs=*/
  Divide_be29b : Product  Inputs=*/
  Divide_c5cfb : Product  Inputs=*/
  Divide_d2884 : Product  Inputs=*/
  Divide_e904c : Product  Inputs=*/
  Product_0f394 : Product
  Product_1a20a : Product
  Product_1c1dd : Product
  Product_20941 : Product
  Product_20d06 : Product
  Product_2277f : Product
  Product_3fb8e : Product
  Product_417fb : Product
  Product_4ebe6 : Product
  Product_4f121 : Product
  Product_594a7 : Product
  Product_5ce64 : Product
  Product_63fef : Product
  Product_66db1 : Product
  Product_86b45 : Product
  Product_8f94b : Product
  Product_9034b : Product
  Product_a567b : Product
  Product_abc7a : Product
  Product_ae3bd : Product
  Product_c11f6 : Product
  Product_e2b3a : Product
  Subtract_038ab : Sum  Inputs=+-
  Subtract_1d341 : Sum  Inputs=+-
  Subtract_30707 : Sum  Inputs=+-
  Subtract_3120a : Sum  Inputs=+-
  Subtract_60887 : Sum  Inputs=+-
  Subtract_afa00 : Sum  Inputs=+-
  Subtract_de12a : Sum  Inputs=+-
  Subtract_e0764 : Sum  Inputs=+-
  Blockout_d_w_SG_D_1_3285d : Outport
  wires:
  Product_0f394/1 -> Add_cc6fe/1
  Constant_-1_7bf97/1 -> Product_86b45/1
  Constant_pi_d3bc3/1 -> Product_abc7a/2
  Constant_x_qdd_b7d14/1 -> Add_0370f/2
  Constant_x_l_b4faa/1 -> Product_86b45/2
  Product_86b45/1 -> Add_0370f/1
  Constant_x_qd_acc8f/1 -> Subtract_30707/1
  Constant_-1_fc7b6/1 -> Product_1a20a/1
  Product_2277f/1 -> Product_0f394/1
  Constant_x_qdd_d8d98/1 -> Subtract_30707/2
  State_psi_q_SG_D_1_cdd53/1 -> Product_ae3bd/1
  Constant_x_l_b32d9/1 -> Product_1a20a/2
  Constant_-1_f811d/1 -> Product_3fb8e/1
  Constant_x_l_5df41/1 -> Product_3fb8e/2
  Constant_-1_bb22b/1 -> Product_20941/1
  Product_1a20a/1 -> Add_d22a5/1
  State_psi_1d_SG_D_1_43d35/1 -> Product_20941/2
  Constant_x_dd_1f675/1 -> Subtract_afa00/1
  Subtract_30707/1 -> Product_66db1/2
  Constant_x_ddd_b94a9/1 -> Subtract_afa00/2
  State_psi_gq_SG_D_1_0a0d0/1 -> Product_417fb/1
  Product_1c1dd/1 -> Product_4f121/1
  Add_0370f/1 -> Product_417fb/2
  Constant_x_qd_e0993/1 -> Add_d22a5/2
  State_psi_kq_SG_D_1_b491e/1 -> Product_66db1/1
  Constant_f0_77ee7/1 -> Product_0f394/2
  Product_3fb8e/1 -> Add_bb789/1
  Constant_x_dd_0d903/1 -> Subtract_e0764/1
  Constant_x_qd_df2e8/1 -> Add_bb789/2
  Product_20941/1 -> Product_20d06/1
  Subtract_afa00/1 -> Product_20d06/2
  Constant_x_l_b2671/1 -> Subtract_e0764/2
  Constant_x_ddd_36e05/1 -> Subtract_3120a/1
  Constant_x_l_2525c/1 -> Subtract_3120a/2
  State_w_SG_D_1_f1fc7/1 -> Add_cc6fe/2
  Divide_22a45/1 -> Add_c220d/1
  Constant_-1_4399d/1 -> Product_4ebe6/1
  Product_417fb/1 -> Divide_d2884/1
  Add_cc6fe/1 -> Product_a567b/2
  Divide_d2884/1 -> Subtract_60887/1
  Add_d22a5/1 -> Divide_d2884/2
  Constant_pi_1e48c/1 -> Product_2277f/2
  Product_66db1/1 -> Divide_502fd/1
  Add_bb789/1 -> Divide_502fd/2
  Product_20d06/1 -> Divide_be29b/1
  Divide_be29b/1 -> Add_14423/1
  Subtract_e0764/1 -> Divide_be29b/2
  State_psi_fd_SG_D_1_f25db/1 -> Product_c11f6/1
  Subtract_3120a/1 -> Product_c11f6/2
  Constant_x_dd_3ac91/1 -> Subtract_038ab/1
  Constant_x_l_fcafc/1 -> Subtract_038ab/2
  Divide_502fd/1 -> Subtract_60887/2
  Constant_2.0_def3d/1 -> Product_abc7a/1
  State_psi_d_SG_D_1_a02c6/1 -> Add_14423/2
  Product_c11f6/1 -> Divide_c5cfb/1
  Subtract_038ab/1 -> Divide_c5cfb/2
  Constant_-2.0_991e3/1 -> Product_2277f/1
  Constant_-1_a6f76/1 -> Product_1c1dd/1
  State_psi_d_SG_D_1_8ac56/1 -> Product_1c1dd/2
  Subtract_60887/1 -> Add_c6f8e/1
  Subtract_de12a/1 -> Product_ae3bd/2
  State_psi_q_SG_D_1_932f1/1 -> Add_c6f8e/2
  Add_14423/1 -> Subtract_de12a/1
  Divide_c5cfb/1 -> Subtract_de12a/2
  Add_c6f8e/1 -> Product_4f121/2
  Constant_D_b2a27/1 -> Product_4ebe6/2
  Product_abc7a/1 -> Product_8f94b/1
  State_T_m_SG_D_1_318e6/1 -> Product_8f94b/2
  Constant_2.0_fc0f9/1 -> Product_63fef/1
  Constant_pi_8a500/1 -> Product_63fef/2
  Product_4f121/1 -> Divide_22a45/1
  Constant_x_qdd_666a9/1 -> Divide_22a45/2
  Product_ae3bd/1 -> Divide_7b2c7/1
  Constant_x_ddd_b90f1/1 -> Divide_7b2c7/2
  Product_4ebe6/1 -> Product_a567b/1
  Product_8f94b/1 -> Product_e2b3a/1
  Constant_f0_d9ea8/1 -> Product_e2b3a/2
  Product_63fef/1 -> Product_9034b/1
  Constant_f0_fed87/1 -> Product_9034b/2
  Divide_7b2c7/1 -> Add_c220d/2
  Product_a567b/1 -> Add_ae8df/1
  Product_e2b3a/1 -> Add_ae8df/2
  Product_9034b/1 -> Product_5ce64/1
  Add_c220d/1 -> Product_5ce64/2
  Add_ae8df/1 -> Subtract_1d341/1
  Product_5ce64/1 -> Subtract_1d341/2
  Constant_2.0_722b3/1 -> Product_594a7/1
  Constant_H_8d1fb/1 -> Product_594a7/2
  Subtract_1d341/1 -> Divide_e904c/1
  Product_594a7/1 -> Divide_e904c/2
  Divide_e904c/1 -> Blockout_d_w_SG_D_1_3285d/1

== system IEEE9_case/SG_D_1/i_d_SG_D_1_block ==
  note: i_d_SG_D_1 in IEEE9_case
      | $\frac{\sin\left(\theta _{\mathrm{SG},D,1}\right)\,\left(\frac{\psi _{\mathrm{1d},\mathrm{SG},D,1}\,\left(x_{\mathrm{dd}}-x_{\mathrm{ddd}}\right)}{x_{\mathrm{dd}}-x_{l}}-\psi _{d,\mathrm{SG},D,1}+\frac{\psi _{\mathrm{fd},\mathrm{SG},D,1}\,\left(x_{\mathrm{ddd}}-x_{l}\right)}{x_{\mathrm{dd}}-x_{l}}\right)}{x_{\mathrm{ddd}}}-\frac{\cos\left(\theta _{\mathrm{SG},D,1}\right)\,\left(\psi _{q,\mathrm{SG},D,1}+\frac{\psi _{\mathrm{gq},\mathrm{SG},D,1}\,\left(x_{l}-x_{\mathrm{qdd}}\right)}{x_{l}-x_{\mathrm{qd}}}+\frac{\psi _{\mathrm{kq},\mathrm{SG},D,1}\,\left(x_{\mathrm{qd}}-x_{\mathrm{qdd}}\right)}{x_{l}-x_{\mathrm{qd}}}\right)}{x_{\mathrm{qdd}}}$
      | Automatically generated on 2025-11-01 08:48:12 .
  State_psi_gq_SG_D_1_953b8 : Inport
  State_psi_kq_SG_D_1_f1a3f : Inport  Port=2
  State_psi_q_SG_D_1_208f7 : Inport  Port=3
  State_theta_SG_D_1_67276 : Inport  Port=4
  State_psi_1d_SG_D_1_26fc3 : Inport  Port=5
  State_psi_d_SG_D_1_a79fb : Inport  Port=6
  State_psi_fd_SG_D_1_19090 : Inport  Port=7
  State_theta_SG_D_1_fdfe6 : Inport  Port=8
  Add_802dc : Sum
  Add_8e2c7 : Sum
  Add_98bf9 : Sum
  Add_a8ab6 : Sum
  Add_f99a3 : Sum
  Constant_-1_50bdb : Constant  Value=-1
  Constant_-1_a8148 : Constant  Value=-1
  Constant_-1_a8e64 : Constant  Value=-1
  Constant_-1_b9f1c : Constant  Value=-1
  Constant_-1_dd788 : Constant  Value=-1
  Constant_x_dd_76ca1 : Constant  Value=x_dd
  Constant_x_dd_af4b1 : Constant  Value=x_dd
  Constant_x_dd_ce5d3 : Constant  Value=x_dd
  Constant_x_ddd_5498f : Constant  Value=x_ddd
  Constant_x_ddd_a1df4 : Constant  Value=x_ddd
  Constant_x_ddd_c3e60 : Constant  Value=x_ddd
  Constant_x_l_03ae5 : Constant  Value=x_l
  Constant_x_l_1879f : Constant  Value=x_l
  Constant_x_l_1a9e4 : Constant  Value=x_l
  Constant_x_l_40817 : Constant  Value=x_l
  Constant_x_l_671e9 : Constant  Value=x_l
  Constant_x_l_f6dbb : Constant  Value=x_l
  Constant_x_qd_2105a : Constant  Value=x_qd
  Constant_x_qd_7b296 : Constant  Value=x_qd
  Constant_x_qd_d33c0 : Constant  Value=x_qd
  Constant_x_qdd_1de65 : Constant  Value=x_qdd
  Constant_x_qdd_2e74f : Constant  Value=x_qdd
  Constant_x_qdd_6a05e : Constant  Value=x_qdd
  Divide_04168 : Product  Inputs=*/
  Divide_193ea : Product  Inputs=*/
  Divide_4164c : Product  Inputs=*/
  Divide_b90ff : Product  Inputs=*/
  Divide_cb59e : Product  Inputs=*/
  Divide_ef703 : Product  Inputs=*/
  MathFunc_cos_af366 : Trigonometry  Operator=cos
  MathFunc_sin_bfb43 : Trigonometry
  Product_0323b : Product
  Product_0c1fb : Product
  Product_1016d : Product
  Product_17fbe : Product
  Product_30456 : Product
  Product_4d4b2 : Product
  Product_734ff : Product
  Product_7b0fe : Product
  Product_8d75b : Product
  Product_a7e36 : Product
  Product_f3a12 : Product
  Subtract_03b14 : Sum  Inputs=+-
  Subtract_3acf4 : Sum  Inputs=+-
  Subtract_693d4 : Sum  Inputs=+-
  Subtract_a2503 : Sum  Inputs=+-
  Subtract_a6338 : Sum  Inputs=+-
  Subtract_d90bc : Sum  Inputs=+-
  Subtract_de79b : Sum  Inputs=+-
  Subtract_f085b : Sum  Inputs=+-
  Blockout_i_d_SG_D_1_09dc5 : Outport
  wires:
  Constant_-1_dd788/1 -> Product_17fbe/1
  Constant_x_l_671e9/1 -> Product_17fbe/2
  Constant_x_ddd_a1df4/1 -> Subtract_03b14/2
  Product_17fbe/1 -> Add_8e2c7/1
  Constant_x_qdd_2e74f/1 -> Subtract_3acf4/2
  Constant_x_l_03ae5/1 -> Product_f3a12/2
  Constant_x_qd_7b296/1 -> Add_a8ab6/2
  Constant_x_qdd_6a05e/1 -> Add_8e2c7/2
  Constant_x_qd_d33c0/1 -> Subtract_3acf4/1
  MathFunc_cos_af366/1 -> Product_7b0fe/2
  Constant_-1_b9f1c/1 -> Product_f3a12/1
  Constant_-1_50bdb/1 -> Product_0c1fb/1
  Subtract_de79b/1 -> Blockout_i_d_SG_D_1_09dc5/1
  Constant_x_l_1a9e4/1 -> Product_0c1fb/2
  Divide_b90ff/1 -> Subtract_693d4/1
  State_psi_gq_SG_D_1_953b8/1 -> Product_a7e36/1
  Subtract_d90bc/1 -> Product_30456/2
  Add_8e2c7/1 -> Product_a7e36/2
  Divide_ef703/1 -> Add_802dc/1
  Product_f3a12/1 -> Add_f99a3/1
  Constant_x_qd_2105a/1 -> Add_f99a3/2
  State_psi_kq_SG_D_1_f1a3f/1 -> Product_8d75b/1
  Add_802dc/1 -> Subtract_f085b/1
  Add_f99a3/1 -> Divide_b90ff/2
  Subtract_3acf4/1 -> Product_8d75b/2
  Product_0c1fb/1 -> Add_a8ab6/1
  Constant_-1_a8148/1 -> Product_0323b/1
  State_psi_1d_SG_D_1_26fc3/1 -> Product_0323b/2
  Constant_x_dd_af4b1/1 -> Subtract_03b14/1
  Product_a7e36/1 -> Divide_b90ff/1
  Product_734ff/1 -> Divide_04168/1
  Subtract_03b14/1 -> Product_1016d/2
  Product_8d75b/1 -> Divide_4164c/1
  Product_0323b/1 -> Product_1016d/1
  Add_a8ab6/1 -> Divide_4164c/2
  Constant_x_dd_ce5d3/1 -> Subtract_a6338/1
  Subtract_693d4/1 -> Add_98bf9/1
  Constant_x_l_f6dbb/1 -> Subtract_a6338/2
  Constant_x_ddd_c3e60/1 -> Subtract_d90bc/1
  Constant_x_l_40817/1 -> Subtract_d90bc/2
  Divide_04168/1 -> Subtract_de79b/2
  Divide_4164c/1 -> Subtract_693d4/2
  State_theta_SG_D_1_67276/1 -> MathFunc_cos_af366/1
  Product_1016d/1 -> Divide_ef703/1
  Subtract_a6338/1 -> Divide_ef703/2
  State_theta_SG_D_1_fdfe6/1 -> MathFunc_sin_bfb43/1
  State_psi_fd_SG_D_1_19090/1 -> Product_30456/1
  Constant_x_dd_76ca1/1 -> Subtract_a2503/1
  Constant_x_l_1879f/1 -> Subtract_a2503/2
  State_psi_q_SG_D_1_208f7/1 -> Add_98bf9/2
  State_psi_d_SG_D_1_a79fb/1 -> Add_802dc/2
  Constant_x_ddd_5498f/1 -> Divide_04168/2
  MathFunc_sin_bfb43/1 -> Product_734ff/2
  Product_30456/1 -> Divide_cb59e/1
  Constant_-1_a8e64/1 -> Product_4d4b2/1
  Subtract_a2503/1 -> Divide_cb59e/2
  Add_98bf9/1 -> Product_4d4b2/2
  Divide_cb59e/1 -> Subtract_f085b/2
  Product_4d4b2/1 -> Product_7b0fe/1
  Subtract_f085b/1 -> Product_734ff/1
  Constant_x_qdd_1de65/1 -> Divide_193ea/2
  Product_7b0fe/1 -> Divide_193ea/1
  Divide_193ea/1 -> Subtract_de79b/1
